simulink model "closedloop"  (Simulink 7.4)
settings: Solver=ode45  StartTime=0.0  StopTime=200  FixedStep=0.05  MaxStep=0.05  RelTol=1e-3
values from neighbouring files (symbols this model uses):
  m = 2    [const_mpc.m]    (also in test_predictions.m)
  Ts = 0.05    [test_linearization.m]    (also in test_observer.m; test_predictions.m)
  ucontrolsize = 2    [const_mpc.m]
  xtotalsize = xsize + 2*sum(n_delay) + 2*dsize    [MpcSetup.m]    (also in get_qp_matrices.m)
libraries: lib_controller x8, dspmtrx3 x6, lib_parallel_comp x1
settings Model: Creator=chkajon  LastModifiedBy=chkajon
settings SFSimCC: SimUserSources=../call_qpoases_m/call_qpoases.c
settings SFSimCC: SimUserIncludeDirs=|
  | ../call_qpoases_m/qpoases3/src
  | ../call_qpoases_m/qpoases3/include

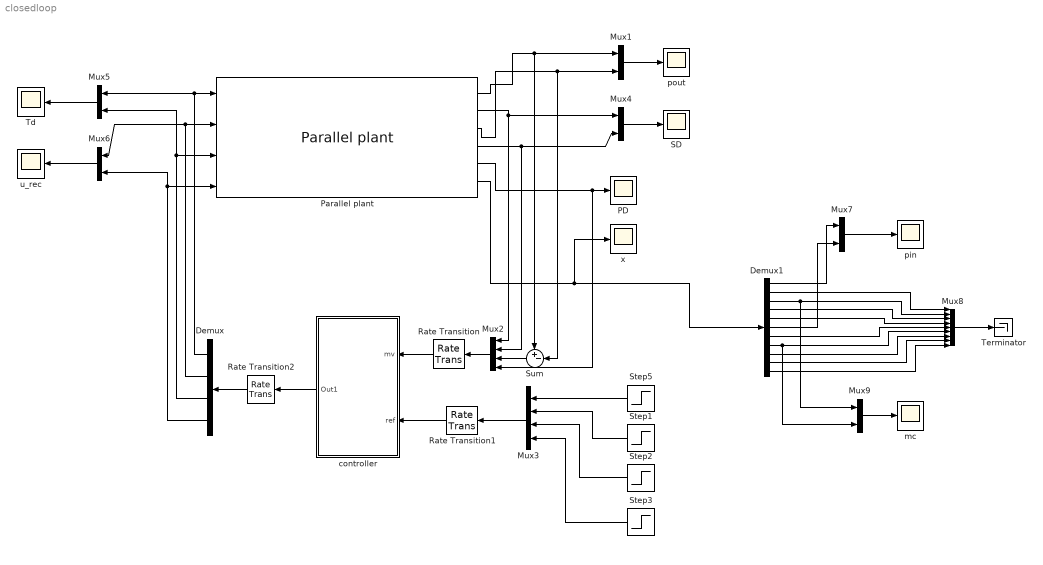
== system closedloop ==
  Demux : Demux
  Demux1 : Demux  Outputs=11
  Mux{1,4..7,9} (6 alike) : Mux  Inputs=2
  Mux2 : Mux
  Mux3 : Mux
  Mux8 : Mux  Inputs=9
  PD : Scope
      settings: TimeRange=100  YMin=1.12  YMax=1.131  SaveName=SD1  DataFormat=Array
  Parallel plant : lib_parallel_comp/Parallel plant  SystemSampleTime=-1  disturbances_on=on  disturbances_symm=on  dist_t=30  dist1=[0 0 -0.2]  dist2=0
  Rate Transition : RateTransition  X0=[0.2;0.2;0;1.08]
  Rate Transition1 : RateTransition
  Rate Transition2 : RateTransition
  SD : Scope
      settings: TimeRange=100  YMin=-0.2  YMax=0.35  SaveName=SD3  DataFormat=Array
  Step1 : Step  Time=0  Before=0.22  After=0.22  SampleTime=0
  Step2 : Step  Time=0  After=0  SampleTime=0
  Step3 : Step  Time=0  Before=1.12  After=1.12  SampleTime=0
  Step5 : Step  Time=0  Before=0.22  After=0.22  SampleTime=0
  Sum : Sum  Inputs=+-|  OutDataType=fixdt(1, 16)  OutScaling=2^0
  Td : Scope
      settings: TimeRange=100  YMin=-0.025  YMax=0.325  SaveName=SD4  DataFormat=Array
  Terminator : Terminator
  controller : Subsystem  TreatAsAtomicUnit=on  SystemSampleTime=Ts
  mc : Scope
      settings: TimeRange=200  YMin=0.1175  YMax=0.155  SaveName=SD8  DataFormat=Array
  pin : Scope
      settings: TimeRange=200  YMin=0.89  YMax=1  SaveName=SD7  DataFormat=Array
  pout : Scope
      settings: TimeRange=100  YMin=-0.07  YMax=0.08  SaveName=SD2  DataFormat=Array
  u_rec : Scope
      settings: TimeRange=100  YMin=0  YMax=0.07  SaveName=SD5  DataFormat=Array
  x : Scope
      settings: TimeRange=85  YMin=1.1125  YMax=1.1141  SaveName=SD6  DataFormat=Array
  wires:
  controller/1(Out1) -> Rate Transition2/1
  Mux2/1 -> Rate Transition/1
  Mux3/1 -> Rate Transition1/1
  Rate Transition/1 -> controller/1(mv)
  Rate Transition1/1 -> controller/2(ref)
  Rate Transition2/1 -> Demux/1
  Demux/1 -> Mux5/1, Parallel plant/1
  Demux/2 -> Mux6/1, Parallel plant/2
  Demux/3 -> Mux5/2, Parallel plant/3
  Demux/4 -> Mux6/2, Parallel plant/4
  Step5/1 -> Mux3/1
  Step1/1 -> Mux3/2
  Step2/1 -> Mux3/3
  Step3/1 -> Mux3/4
  Parallel plant/1 -> Mux1/1, Sum/1
  Parallel plant/5 -> PD/1, Mux2/4
  Parallel plant/2 -> Mux4/1, Mux2/1
  Parallel plant/3 -> Mux1/2, Sum/2
  Mux4/1 -> SD/1
  Mux1/1 -> pout/1
  Mux5/1 -> Td/1
  Mux6/1 -> u_rec/1
  Parallel plant/6 -> x/1, Demux1/1
  Demux1/1 -> Mux7/1
  Demux1/6 -> Mux7/2
  Demux1/2 -> Mux8/1
  Demux1/3 -> Mux8/2, Mux9/1
  Demux1/4 -> Mux8/3
  Demux1/5 -> Mux8/4
  Demux1/7 -> Mux8/5
  Demux1/8 -> Mux8/6, Mux9/2
  Demux1/9 -> Mux8/7
  Demux1/10 -> Mux8/8
  Demux1/11 -> Mux8/9
  Mux8/1 -> Terminator/1
  Mux7/1 -> pin/1
  Mux9/1 -> mc/1
  Sum/1 -> Mux2/3
  Parallel plant/4 -> Mux4/2, Mux2/2

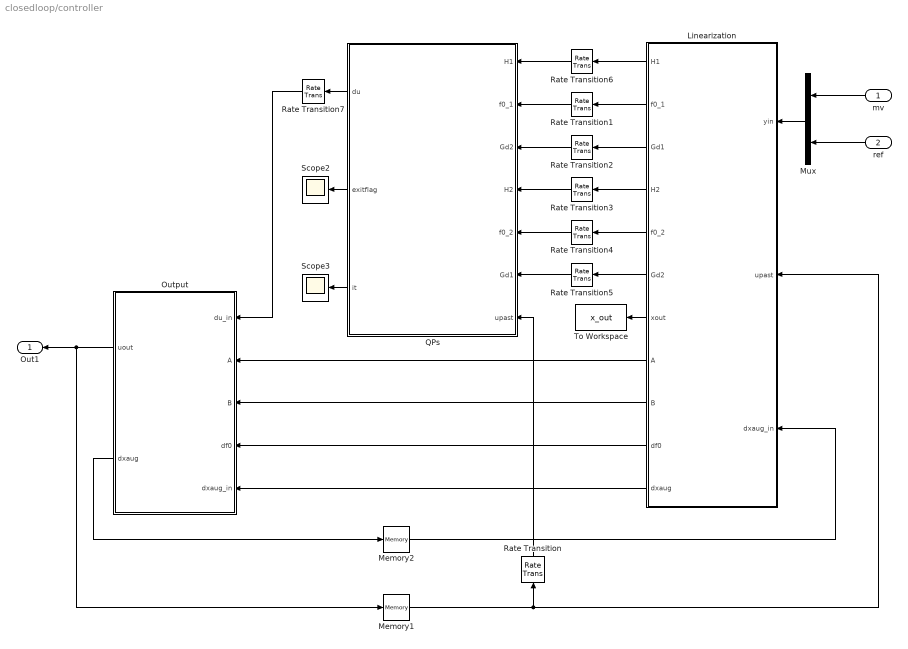
== system closedloop/controller ==
  mv : Inport
  ref : Inport  Port=2
  Linearization : Stateflow chart  SystemSampleTime=Ts
  Memory1 : Memory  X0=zeros(2*ucontrolsize,1)  InheritSampleTime=on
  Memory2 : Memory  X0=zeros(xtotalsize,1)  InheritSampleTime=on
  Mux : Mux  Inputs=2
  Output : Stateflow chart  SystemSampleTime=Ts
  QPs : Subsystem  SystemSampleTime=Ts/3
  Rate Transition : RateTransition  X0=zeros(2*ucontrolsize,1)
  Rate Transition{1..7} (7 alike) : RateTransition
  Scope2 : Scope
      settings: YMin=-1  YMax=1  SaveName=ScopeData15
  Scope3 : Scope
      settings: YMin=10  YMax=47.5  SaveName=ScopeData16
  To Workspace : ToWorkspace  VariableName=x_out  SampleTime=-1  SaveFormat=Structure With Time
  Out1 : Outport
  wires:
  mv/1 -> Mux/1
  ref/1 -> Mux/2
  Memory1/1 -> Linearization/2(upast), Rate Transition/1
  Memory2/1 -> Linearization/3(dxaug_in)
  Output/1(uout) -> Memory1/1, Out1/1
  Output/2(dxaug) -> Memory2/1
  QPs/1(du) -> Rate Transition7/1
  Linearization/7(xout) -> To Workspace/1
  QPs/2(exitflag) -> Scope2/1
  QPs/3(it) -> Scope3/1
  Linearization/8(A) -> Output/2(A)
  Linearization/9(B) -> Output/3(B)
  Linearization/10(df0) -> Output/4(df0)
  Linearization/11(dxaug) -> Output/5(dxaug_in)
  Rate Transition/1 -> QPs/7(upast)
  Linearization/1(H1) -> Rate Transition6/1
  Rate Transition6/1 -> QPs/1(H1)
  Linearization/2(f0_1) -> Rate Transition1/1
  Rate Transition1/1 -> QPs/2(f0_1)
  Linearization/3(Gd1) -> Rate Transition2/1
  Linearization/4(H2) -> Rate Transition3/1
  Linearization/5(f0_2) -> Rate Transition4/1
  Linearization/6(Gd2) -> Rate Transition5/1
  Rate Transition2/1 -> QPs/3(Gd2)
  Rate Transition3/1 -> QPs/4(H2)
  Rate Transition4/1 -> QPs/5(f0_2)
  Rate Transition5/1 -> QPs/6(Gd1)
  Mux/1 -> Linearization/1(yin)
  Rate Transition7/1 -> Output/1(du_in)

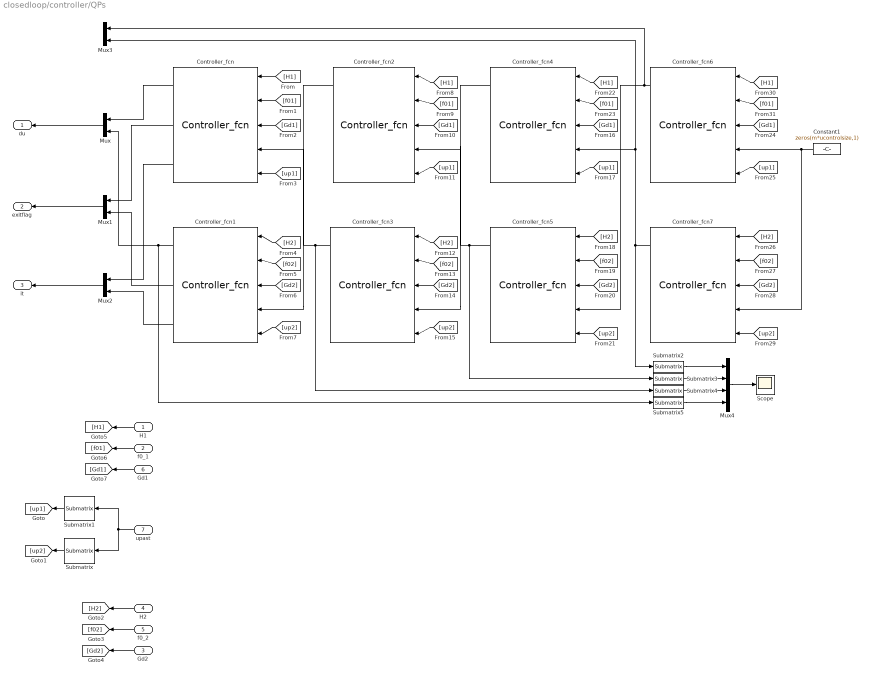
== system closedloop/controller/QPs ==
  H1 : Inport  OutDataType=fixdt(1, 16)  OutScaling=2^0
  f0_1 : Inport  Port=2  OutDataType=fixdt(1, 16)  OutScaling=2^0
  Gd2 : Inport  Port=3  OutDataType=fixdt(1, 16)  OutScaling=2^0
  H2 : Inport  Port=4  OutDataType=fixdt(1, 16)  OutScaling=2^0
  f0_2 : Inport  Port=5  OutDataType=fixdt(1, 16)  OutScaling=2^0
  Gd1 : Inport  Port=6  OutDataType=fixdt(1, 16)  OutScaling=2^0
  upast : Inport  Port=7  OutDataType=fixdt(1, 16)  OutScaling=2^0
  Constant1 : Constant  Value=zeros(m*ucontrolsize,1)  OutDataType=fixdt(1, 16)  OutScaling=2^0  SampleTime=-1
  Controller_fcn{,1..7} (8 alike) : lib_controller/Controller_fcn  SystemSampleTime=-1
  Mux{,1..3} (4 alike) : Mux  Inputs=2
  Mux4 : Mux
  Scope : Scope
      settings: YMin=-0.0011  YMax=0.0007  SaveName=ScopeData4
  Submatrix : dspmtrx3/Submatrix  RowSpan=Range of rows  RowStartMode=Offset from last  RowStartIndex=ucontrolsize-1  RowEndMode=Last  RowEndIndex=2  ColSpan=Range of columns  ColStartMode=First  ColStartIndex=1  ColEndMode=Last  ColEndIndex=2
  Submatrix1 : dspmtrx3/Submatrix  RowSpan=Range of rows  RowStartMode=First  RowStartIndex=1  RowEndMode=Index  RowEndIndex=ucontrolsize  ColSpan=Range of columns  ColStartMode=First  ColStartIndex=1  ColEndMode=Last  ColEndIndex=2
  Submatrix{2..5} (4 alike) : dspmtrx3/Submatrix  RowSpan=Range of rows  RowStartMode=First  RowStartIndex=1  RowEndMode=Index  RowEndIndex=1  ColSpan=Range of columns  ColStartMode=First  ColStartIndex=1  ColEndMode=Index  ColEndIndex=1
  du : Outport  OutDataType=fixdt(1, 16)  OutScaling=2^0
  exitflag : Outport  Port=2  OutDataType=fixdt(1, 16)  OutScaling=2^0
  it : Outport  Port=3  OutDataType=fixdt(1, 16)  OutScaling=2^0
  wires:
  Mux1/1 -> exitflag/1
  Mux2/1 -> it/1
  Controller_fcn/2 -> Mux1/1
  Controller_fcn1/2 -> Mux1/2
  upast/1 -> Submatrix1/1, Submatrix/1
  Submatrix1/1 -> [up1]
  H1/1 -> [H1]
  f0_1/1 -> [f01]
  Gd1/1 -> [Gd1]
  H2/1 -> [H2]
  f0_2/1 -> [f02]
  Gd2/1 -> [Gd2]
  Submatrix/1 -> [up2]
  Controller_fcn1/3 -> Mux2/2
  Controller_fcn1/1 -> Mux/2, Submatrix5/1
  Controller_fcn/1 -> Mux/1
  Controller_fcn/3 -> Mux2/1
  [H1] -> Controller_fcn/1
  [f01] -> Controller_fcn/2
  [Gd1] -> Controller_fcn/3
  [up1] -> Controller_fcn/5
  [H2] -> Controller_fcn1/1
  [f02] -> Controller_fcn1/2
  [Gd2] -> Controller_fcn1/3
  [up2] -> Controller_fcn1/5
  [H1] -> Controller_fcn2/1
  [f01] -> Controller_fcn2/2
  [Gd1] -> Controller_fcn2/3
  [up1] -> Controller_fcn2/5
  [H2] -> Controller_fcn3/1
  [f02] -> Controller_fcn3/2
  [Gd2] -> Controller_fcn3/3
  [up2] -> Controller_fcn3/5
  [up2] -> Controller_fcn5/5
  [Gd2] -> Controller_fcn5/3
  [f02] -> Controller_fcn5/2
  [up1] -> Controller_fcn4/5
  [Gd1] -> Controller_fcn4/3
  [f01] -> Controller_fcn4/2
  Controller_fcn4/1 -> Controller_fcn3/4
  Controller_fcn5/1 -> Controller_fcn2/4, Submatrix3/1
  Controller_fcn2/1 -> Controller_fcn1/4
  Controller_fcn3/1 -> Controller_fcn/4, Submatrix4/1
  Mux4/1 -> Scope/1
  Submatrix2/1 -> Mux4/1
  Submatrix3/1 -> Mux4/2
  Submatrix4/1 -> Mux4/3
  [H2] -> Controller_fcn5/1
  [H1] -> Controller_fcn4/1
  [up2] -> Controller_fcn7/5
  [Gd2] -> Controller_fcn7/3
  [f02] -> Controller_fcn7/2
  [up1] -> Controller_fcn6/5
  [Gd1] -> Controller_fcn6/3
  [f01] -> Controller_fcn6/2
  Constant1/1 -> Controller_fcn7/4, Controller_fcn6/4
  [H2] -> Controller_fcn7/1
  [H1] -> Controller_fcn6/1
  Controller_fcn6/1 -> Controller_fcn5/4, Mux3/1
  Controller_fcn7/1 -> Submatrix2/1, Controller_fcn4/4, Mux3/2
  Submatrix5/1 -> Mux4/4
  Mux/1 -> du/1

== matlab function controller/Output ==
  data: du_in input double; A input double; B input double; df0 input double; uout output double; dxaug_in input double; dxaug output double
function [uout,dxaug]  = fcn(du_in, A, B, df0, dxaug_in)
%#eml
persistent upast
eml.extrinsic('disp');
eml.extrinsic('toc');
eml.extrinsic('tic');
eml.extrinsic('num2str');
eml.extrinsic('keyboard');
eml.extrinsic('quadprog');



[~, ~, xsize, ~, ~] = const_sim();
[n_delay,~,ucontrolsize,~,m] = const_mpc();

if isempty(upast)
    tic
    upast = zeros(ucontrolsize*2,1);
    time = toc;
    disp(['Preparation time: ' num2str(time)]);
end

% take only the first move from du
du = [du_in(1:ucontrolsize,1); du_in(1+m*ucontrolsize:(m+1)*ucontrolsize,1)];

% Apply next input
u_new = upast + du;

% value of x about which we linearized
xlin = dxaug_in;
xlin(xsize+1:end) = 0;
xlin(xsize+1) = upast(2);
xlin(xsize+1+n_delay(2)) = upast(4);

dxaug = B*[u_new(1)-upast(1);u_new(2);u_new(3)-upast(3);u_new(4)] + A*(dxaug_in-xlin) + df0;

upast = u_new;
uout = u_new;

== matlab function controller/Linearization ==
  data: yin input double; H1 output double; f0_1 output double; Gd1 output double; H2 output double; f0_2 output double; Gd2 output double; xout output double; A output double; B output double; df0 output double; dxaug output double; upast input double; dxaug_in input double
function [H1, f0_1, Gd1, H2, f0_2, Gd2, xout, A, B, df0, dxaug]  = fcn(yin, upast, dxaug_in)
%#eml
% persistent C_new M LB UB Ga Gb Gc H Ain b A B upast xinit
persistent M xinit y_old C 
eml.extrinsic('disp');
eml.extrinsic('toc');
eml.extrinsic('tic');
eml.extrinsic('num2str');
eml.extrinsic('keyboard');
eml.extrinsic('quadprog');



[~, ~, xsize, ~, ysize] = const_sim();
[n_delay,dsize,~,p] = const_mpc();

if isempty(M)
    tic
    [C,M,~,~,~,~,xinit] = get_constant_matrices();
%     y_old = zeros(ysize,1);
    y_old = [0.2175; 0.2175; 0; 1.12];
    time = toc;
    disp(['Preparation time: ' num2str(time)]);
end


y = yin(1:ysize);
yref = yin(ysize+1:end);

% Estimate state info
dxaug = dxaug_in + M*(y - y_old - C*(dxaug_in));

% Use state input info to calculate x, y
xinit(1:xsize) = xinit(1:xsize)+dxaug(1:xsize);
xinit(xsize+1:end) = dxaug(xsize+1:end);

xout = xinit;

% get matrices
[A,B,C,df0,H1,H2,f0_1,f0_2,Gd1,Gd2] = get_qp_matrices(xinit,upast,yref-y);
